simulink model "V3_Modell"  (R2022a)
settings: Solver=ode3  StartTime=0.0  StopTime=Zeit(end)  FixedStep=0.001  RelTol=1e-3
values from neighbouring files (symbols this model uses):
  den = [L_A R_A]    [V3_Parameter.m]
  g = 9.81    [V3_Parameter.m]
  i_G = 62    [V3_Parameter.m]
  J = J_M * (i_G)^2 + J_S + m_G * (r_S)^2    (= 0.23442)    [V3_Parameter.m]
  k_M = 0.107646    [V3_Parameter.m]
  KL_REIB = [-2.32446  -1.72725  -1.14312  -0.55627  -0.001   0  0.001    0.296462  0.893574  1.47885  2.07879 ... (first row only)    [V3_Parameter.m]
  m_G = 2    [V3_Parameter.m]
  num = [1]    [V3_Parameter.m]
  r_S = 0.1    [V3_Parameter.m]
settings Model: Creator=bornkessel  LastModifiedBy=bornk

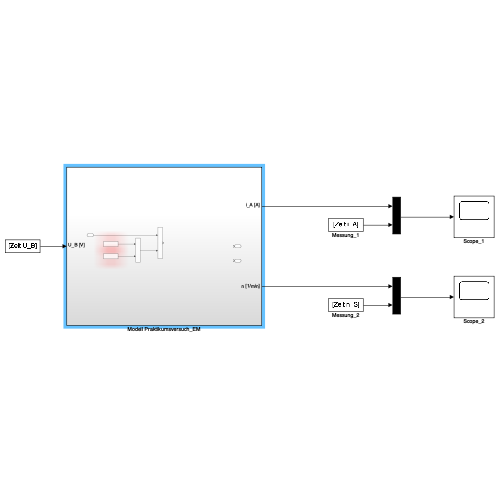
[thumbnail: Simulink's stored preview of the top-level diagram]
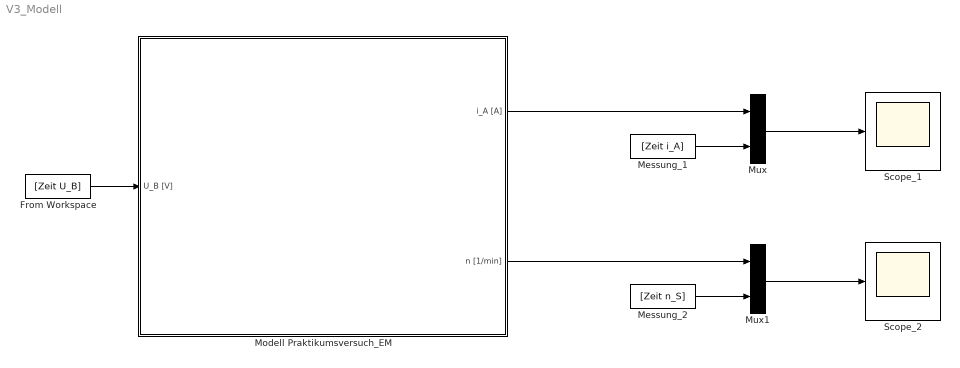
== system V3_Modell ==
  From Workspace : FromWorkspace  VariableName=[Zeit U_B]
  Messung_1 : FromWorkspace  VariableName=[Zeit i_A]
  Messung_2 : FromWorkspace  VariableName=[Zeit n_S]
  Modell Praktikumsversuch_EM : Subsystem
  Mux : Mux  Inputs=2
  Mux1 : Mux  Inputs=2
  Scope_1 : Scope
  Scope_2 : Scope
  wires:
  From Workspace/1 -> Modell Praktikumsversuch_EM/1(U_B [V])
  Modell Praktikumsversuch_EM/1(i_A [A]) -> Mux/1
  Modell Praktikumsversuch_EM/2(n [1/min]) -> Mux1/1
  Messung_1/1 -> Mux/2
  Messung_2/1 -> Mux1/2
  Mux/1 -> Scope_1/1
  Mux1/1 -> Scope_2/1

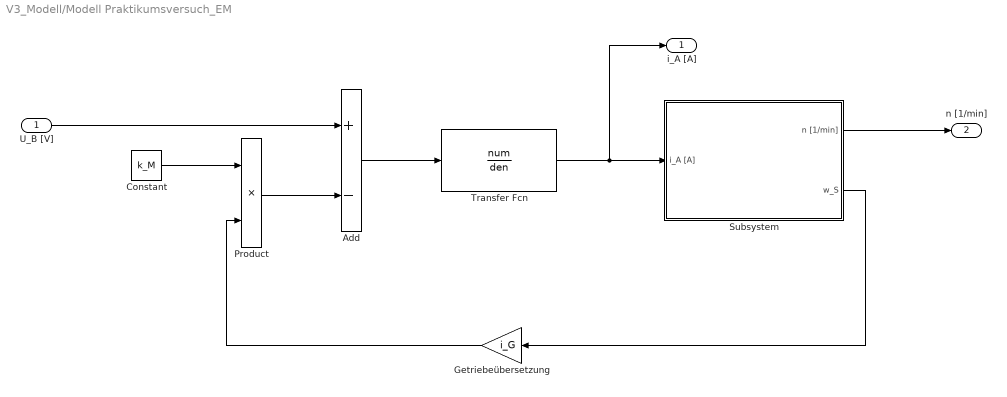
== system V3_Modell/Modell Praktikumsversuch_EM ==
  U_B [V] : Inport
  Add : Sum  Inputs=+-
  Constant : Constant  Value=k_M
  Getriebeübersetzung : Gain  Gain=i_G
  Product : Product
  Subsystem : Subsystem
  Transfer Fcn : TransferFcn  Numerator=num  Denominator=den
  i_A [A] : Outport
  n [1/min] : Outport  Port=2
  wires:
  U_B [V]/1 -> Add/1
  Product/1 -> Add/2
  Constant/1 -> Product/1
  Getriebeübersetzung/1 -> Product/2
  Add/1 -> Transfer Fcn/1
  Transfer Fcn/1 -> i_A [A]/1, Subsystem/1(i_A [A])
  Subsystem/1(n [1/min]) -> n [1/min]/1
  Subsystem/2(w_S) -> Getriebeübersetzung/1

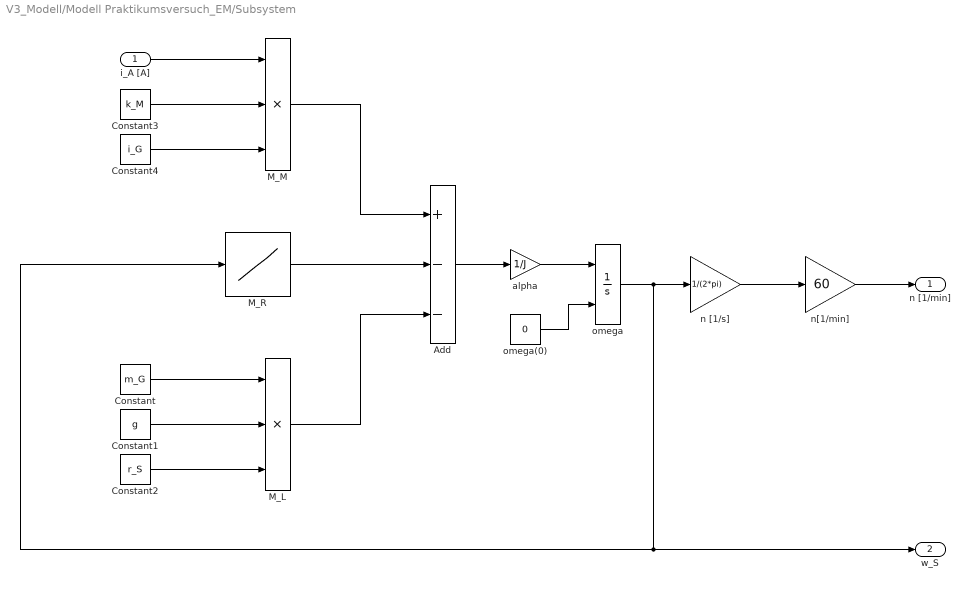
== system V3_Modell/Modell Praktikumsversuch_EM/Subsystem ==
  i_A [A] : Inport
  Add : Sum  Inputs=+--
  Constant : Constant  Value=m_G
  Constant1 : Constant  Value=g
  Constant2 : Constant  Value=r_S
  Constant3 : Constant  Value=k_M
  Constant4 : Constant  Value=i_G
  M_L : Product  Inputs=3
  M_M : Product  Inputs=3
  M_R : Lookup_n-D  NumberOfTableDimensions=1  BreakpointsForDimension1=KL_REIB(1,:)  Table=KL_REIB(2,:)  InternalRulePriority=Speed  RndMeth=Simplest
  alpha : Gain  Gain=1/J
  n [1/s] : Gain  Gain=1/(2*pi)
  n[1/min] : Gain  Gain=60
  omega : Integrator  InitialConditionSource=external
  omega(0) : Constant  Value=0
  n [1/min] : Outport
  w_S : Outport  Port=2
  wires:
  i_A [A]/1 -> M_M/1
  Constant3/1 -> M_M/2
  Constant4/1 -> M_M/3
  Constant/1 -> M_L/1
  Constant1/1 -> M_L/2
  Constant2/1 -> M_L/3
  M_L/1 -> Add/3
  M_M/1 -> Add/1
  Add/1 -> alpha/1
  alpha/1 -> omega/1
  omega/1 -> w_S/1, M_R/1, n [1/s]/1
  n [1/s]/1 -> n[1/min]/1
  n[1/min]/1 -> n [1/min]/1
  omega(0)/1 -> omega/2
  M_R/1 -> Add/2
